simulink model "MeUn_Rot"  (R2016b)
settings: configuration reference "CodeGenConfigSet" (kept outside this file)
values from neighbouring files (symbols this model uses):
  MeUn_ctRot_C = Calibration.Parameter    [init_MeUn_Rot.m]
  MeUn_rLin_CUR = Calibration.Parameter    [init_MeUn_Rot.m]
  MeUn_rLin_CURX = Calibration.Parameter    [init_MeUn_Rot.m]
  MeUn_rRotEnd_C = Calibration.Parameter    [init_MeUn_Rot.m]
  MeUn_rRotStrt_C = Calibration.Parameter    [init_MeUn_Rot.m]
  MeUn_stRotActv_C = Calibration.Parameter    [init_MeUn_Rot.m]
  MeUn_tiRotDel_C = Calibration.Parameter    [init_MeUn_Rot.m]
  MeUn_tiRotWait_C = Calibration.Parameter    [init_MeUn_Rot.m]
undefined symbols (not defined in the file or in its folder): EngState_conv, MeUn_Rot_DT
libraries: CXLib x3
settings Model: Creator=Wollf  LastModifiedBy=mayongchao
settings ConfigSetRef: SourceLocation=Base Workspace

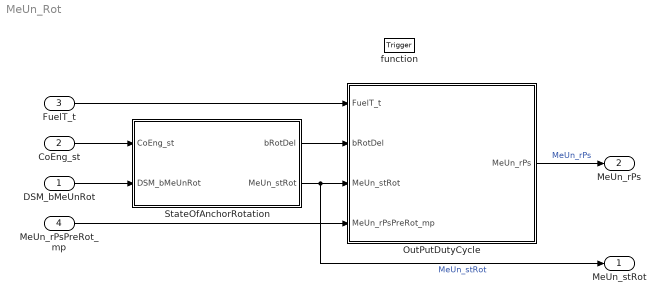
== system MeUn_Rot ==
  DSM_bMeUnRot : Inport  Description=state of FId_MeUnRot  OutMin=0  OutMax=1  OutDataTypeStr=boolean
  CoEng_st : Inport  Description=Engine coordinator state  Port=2  OutDataTypeStr=Enum: EngState_conv
  FuelT_t : Inport  Tag=deg  Description=Temperature of fuel  Port=3  OutMin=-50  OutMax=150  OutDataTypeStr=Temp_deg
  MeUn_rPsPreRot_mp : Inport  Tag=%  Description=duty cycle of meun current governor before rotation  Port=4  OutMin=0  OutMax=100  OutDataTypeStr=DutyCycle_rate
  function : TriggerPort  TriggerType=function-call  VariantControl=Variant
  OutPutDutyCycle : Subsystem
  StateOfAnchorRotation : Subsystem
  MeUn_stRot : Outport  Description=State of anchor rotation function of metering unit  OutMin=0  OutMax=1  OutDataTypeStr=boolean
  MeUn_rPs : Outport  Tag=%  Description=PWM signal output from the metering unit  Port=2  OutMin=0  OutMax=100  OutDataTypeStr=DutyCycle_rate
  wires:
  CoEng_st/1 -> StateOfAnchorRotation/1(CoEng_st)
  DSM_bMeUnRot/1 -> StateOfAnchorRotation/2("DSM_bMeUnRot ")
  MeUn_rPsPreRot_mp/1 -> OutPutDutyCycle/4(MeUn_rPsPreRot_mp)
  OutPutDutyCycle/1(MeUn_rPs) -> MeUn_rPs/1  "MeUn_rPs"
  StateOfAnchorRotation/2(MeUn_stRot) -> MeUn_stRot/1, OutPutDutyCycle/3(MeUn_stRot)  "MeUn_stRot"
  StateOfAnchorRotation/1(bRotDel) -> OutPutDutyCycle/2(bRotDel)
  FuelT_t/1 -> OutPutDutyCycle/1(FuelT_t)

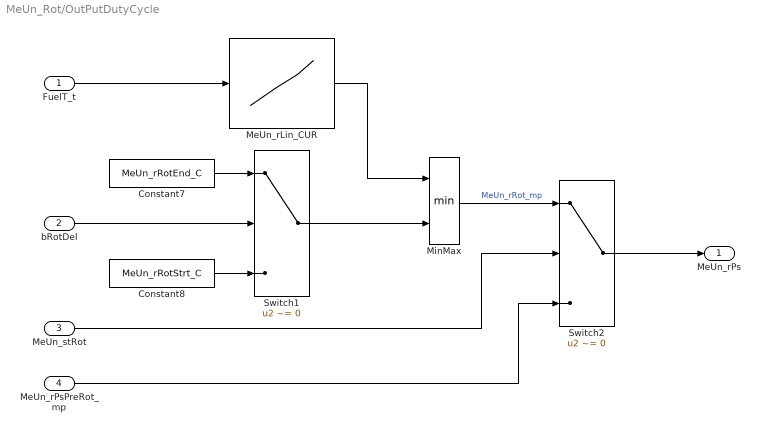
== system MeUn_Rot/OutPutDutyCycle ==
  FuelT_t : Inport
  bRotDel : Inport  Port=2
  MeUn_stRot : Inport  Port=3
  MeUn_rPsPreRot_mp : Inport  Port=4
  Constant7 : Constant  Value=MeUn_rRotEnd_C
  Constant8 : Constant  Value=MeUn_rRotStrt_C
  MeUn_rLin_CUR : Lookup_n-D  NumberOfTableDimensions=1  BreakpointsForDimension1=MeUn_rLin_CURX  IndexSearchMethod=Linear search  BeginIndexSearchUsingPreviousIndexResult=on  Table=MeUn_rLin_CUR  ExtrapMethod=Clip  UseLastTableValue=on  InternalRulePriority=Speed  OutDataTypeStr=Inherit: Inherit via back propagation  SaturateOnIntegerOverflow=on
  MinMax : MinMax  Inputs=2  InputSameDT=on
  Switch1 : Switch  Criteria=u2 ~= 0  InputSameDT=on
  Switch2 : Switch  Criteria=u2 ~= 0  InputSameDT=on
  MeUn_rPs : Outport
  wires:
  MeUn_stRot/1 -> Switch2/2
  bRotDel/1 -> Switch1/2
  MinMax/1 -> Switch2/1  "MeUn_rRot_mp"
  FuelT_t/1 -> MeUn_rLin_CUR/1
  MeUn_rLin_CUR/1 -> MinMax/1
  Switch1/1 -> MinMax/2
  Constant7/1 -> Switch1/1
  Constant8/1 -> Switch1/3
  MeUn_rPsPreRot_mp/1 -> Switch2/3
  Switch2/1 -> MeUn_rPs/1

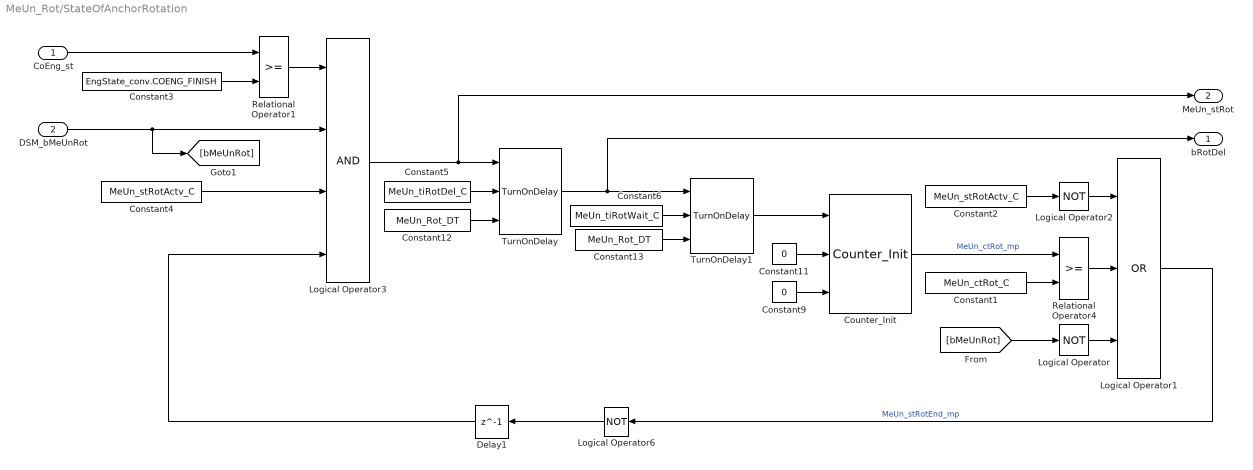
== system MeUn_Rot/StateOfAnchorRotation ==
  CoEng_st : Inport
  "DSM_bMeUnRot " : Inport  Port=2
  Constant1 : Constant  Value=MeUn_ctRot_C
  Constant11 : Constant  Value=0  OutDataTypeStr=Inherit: Inherit via back propagation
  Constant12 : Constant  Value=MeUn_Rot_DT  OutDataTypeStr=Debounce_ms
  Constant13 : Constant  Value=MeUn_Rot_DT  OutDataTypeStr=Debounce_ms
  Constant2 : Constant  Value=MeUn_stRotActv_C
  Constant3 : Constant  Value=EngState_conv.COENG_FINISH  OutDataTypeStr=Inherit: Inherit via back propagation
  Constant4 : Constant  Value=MeUn_stRotActv_C
  Constant5 : Constant  Value=MeUn_tiRotDel_C
  Constant6 : Constant  Value=MeUn_tiRotWait_C
  Constant9 : Constant  Value=0  OutDataTypeStr=Inherit: Inherit via back propagation
  Counter_Init : CXLib/Counter_Init
  Delay1 : Delay  DelayLength=1  InitialCondition=0
  Logical Operator : Logic  Operator=NOT  AllPortsSameDT=off  OutDataTypeStr=boolean
  Logical Operator1 : Logic  Operator=OR  Inputs=3  OutDataTypeStr=boolean
  Logical Operator2 : Logic  Operator=NOT  Inputs=3  AllPortsSameDT=off  OutDataTypeStr=boolean
  Logical Operator3 : Logic  Inputs=4  OutDataTypeStr=boolean
  Logical Operator6 : Logic  Operator=NOT  Inputs=3  AllPortsSameDT=off  OutDataTypeStr=boolean
  Relational Operator1 : RelationalOperator  OutDataTypeStr=boolean  RndMeth=Nearest  InputSameDT=on
  Relational Operator4 : RelationalOperator  OutDataTypeStr=boolean  RndMeth=Nearest  InputSameDT=on
  TurnOnDelay : CXLib/TurnOnDelay
  TurnOnDelay1 : CXLib/TurnOnDelay
  bRotDel : Outport
  MeUn_stRot : Outport  Port=2
  wires:
  Constant1/1 -> Relational Operator4/2
  Counter_Init/1 -> Relational Operator4/1  "MeUn_ctRot_mp"
  Constant2/1 -> Logical Operator2/1
  [bMeUnRot] -> Logical Operator/1
  CoEng_st/1 -> Relational Operator1/1
  Relational Operator1/1 -> Logical Operator3/1
  "DSM_bMeUnRot "/1 -> [bMeUnRot], Logical Operator3/2
  Delay1/1 -> Logical Operator3/4
  TurnOnDelay/1 -> TurnOnDelay1/1, bRotDel/1
  TurnOnDelay1/1 -> Counter_Init/1
  Logical Operator6/1 -> Delay1/1
  Constant3/1 -> Relational Operator1/2
  Constant4/1 -> Logical Operator3/3
  Constant5/1 -> TurnOnDelay/2
  Constant6/1 -> TurnOnDelay1/2
  Logical Operator1/1 -> Logical Operator6/1  "MeUn_stRotEnd_mp"
  Constant9/1 -> Counter_Init/3
  Constant11/1 -> Counter_Init/2
  Constant12/1 -> TurnOnDelay/3
  Constant13/1 -> TurnOnDelay1/3
  Logical Operator2/1 -> Logical Operator1/1
  Relational Operator4/1 -> Logical Operator1/2
  Logical Operator/1 -> Logical Operator1/3
  Logical Operator3/1 -> MeUn_stRot/1, TurnOnDelay/1
